simulink model "controlSystem"  (R2017a)
settings: Solver=VariableStepAuto  StartTime=0.0  StopTime=2  MaxStep=0.01  RelTol=1e-4  EnableMultiTasking=on
model workspace (MAT data in the model file):
  matrix = Simulink.Parameter
  matrix.DataType = 'auto'
  matrix.Dimensions = [0 0]
settings Model: Creator=se_marc  LastModifiedBy=se_marc
settings SolverCC: MaxConsecutiveMinStep=100
settings DataIOCC: LimitDataPoints=on  SaveOutput=off  SaveTime=off
settings OptimizationCC: ExpressionDepthLimit=2147483647  LifeSpan=1
settings DebuggingCC: UnderspecifiedInitializationDetection=Classic  MergeDetectMultiDrivingBlocksExec=none  FcnCallInpInsideContextMsg=warning  AllowSymbolicDim=off  StateNameClashWarn=warning  SFUnexpectedBacktrackingDiag=warning  SFNoUnconditionalDefaultTransitionDiag=warning  SFExecutionAtInitializationDiag=none
settings GRTTargetCC: TargetLangStandard=C89/C90 (ANSI)  GeneratePreprocessorConditionals=Disable all  CombineOutputUpdateFcns=off  GRTInterface=on

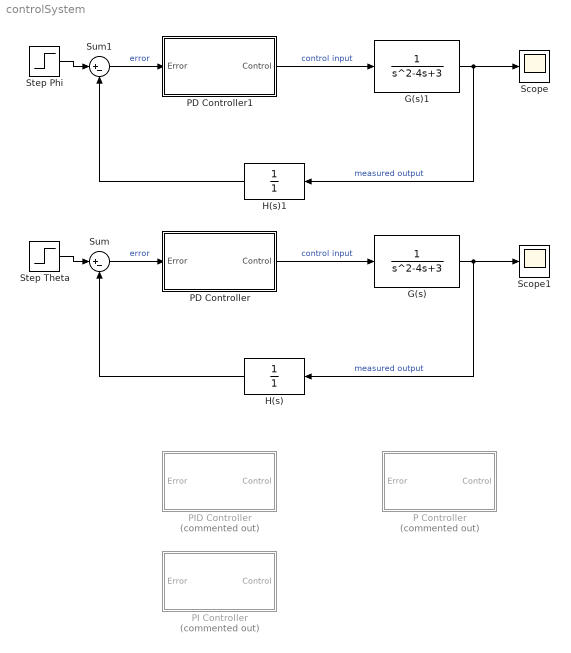
== system controlSystem ==
  G(s) : TransferFcn  Numerator=1  Denominator=[1 -4 3]
  G(s)1 : TransferFcn  Numerator=1  Denominator=[1 -4 3]
  H(s) : TransferFcn  Denominator=[1]
  H(s)1 : TransferFcn  Denominator=[1]
  P Controller : Subsystem  Commented=on
  PD Controller : Subsystem
  PD Controller1 : Subsystem
  PI Controller : Subsystem  Commented=on
  PID Controller : Subsystem  Commented=on
  Scope : Scope
  Scope1 : Scope
  Step Phi : Step  Before=0.034907  After=0.087266  SampleTime=0
  Step Theta : Step  Before=1.4661  After=-1.1519  SampleTime=0
  Sum : Sum  Inputs=|+-
  Sum1 : Sum  Inputs=|+-
  wires:
  G(s)/1 -> Scope1/1, H(s)/1  "measured output"
  Sum/1 -> PD Controller/1(Error)  "error"
  PD Controller/1(Control) -> G(s)/1  "control input"
  H(s)/1 -> Sum/2
  Step Theta/1 -> Sum/1
  Step Phi/1 -> Sum1/1
  Sum1/1 -> PD Controller1/1(Error)  "error"
  G(s)1/1 -> Scope/1, H(s)1/1  "measured output"
  PD Controller1/1(Control) -> G(s)1/1  "control input"
  H(s)1/1 -> Sum1/2

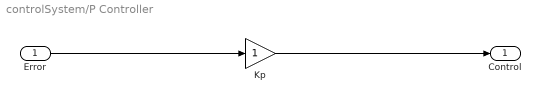
== system controlSystem/P Controller ==
  Error : Inport
  Kp : Gain
  Control : Outport
  wires:
  Error/1 -> Kp/1
  Kp/1 -> Control/1

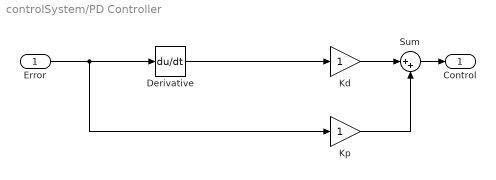
== system controlSystem/PD Controller ==
  Error : Inport
  Derivative : Derivative
  Kd : Gain
  Kp : Gain
  Sum : Sum  Inputs=|++
  Control : Outport
  wires:
  Error/1 -> Derivative/1, Kp/1
  Derivative/1 -> Kd/1
  Kp/1 -> Sum/2
  Sum/1 -> Control/1
  Kd/1 -> Sum/1

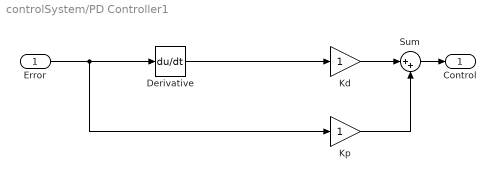
== system controlSystem/PD Controller1 ==
  Error : Inport
  Derivative : Derivative
  Kd : Gain
  Kp : Gain
  Sum : Sum  Inputs=|++
  Control : Outport
  wires:
  Error/1 -> Derivative/1, Kp/1
  Derivative/1 -> Kd/1
  Kp/1 -> Sum/2
  Sum/1 -> Control/1
  Kd/1 -> Sum/1

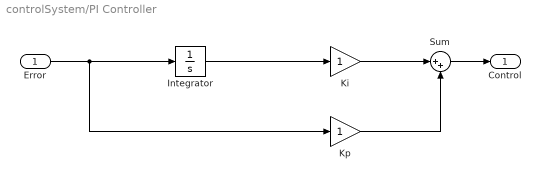
== system controlSystem/PI Controller ==
  Error : Inport
  Integrator : Integrator
  Ki : Gain
  Kp : Gain
  Sum : Sum  Inputs=|++
  Control : Outport
  wires:
  Error/1 -> Integrator/1, Kp/1
  Kp/1 -> Sum/2
  Sum/1 -> Control/1
  Integrator/1 -> Ki/1
  Ki/1 -> Sum/1

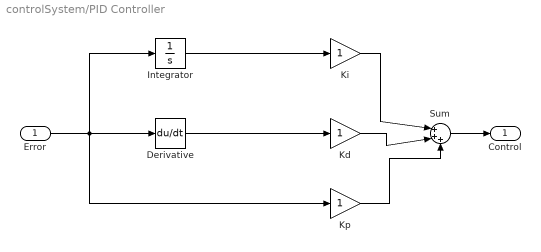
== system controlSystem/PID Controller ==
  Error : Inport
  Derivative : Derivative
  Integrator : Integrator
  Kd : Gain
  Ki : Gain
  Kp : Gain
  Sum : Sum  Inputs=|+++
  Control : Outport
  wires:
  Error/1 -> Integrator/1, Derivative/1, Kp/1
  Derivative/1 -> Kd/1
  Kp/1 -> Sum/3
  Sum/1 -> Control/1
  Kd/1 -> Sum/2
  Integrator/1 -> Ki/1
  Ki/1 -> Sum/1
